simulink model "callZumoExtrinsic_runMotors"  (R2014a)
settings: Solver=FixedStepDiscrete  StartTime=0.0  StopTime=inf  FixedStep=0.1  RelTol=1e-3
settings Model: Creator=nrattner  LastModifiedBy=sandip

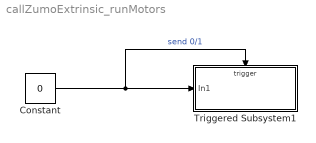
== system callZumoExtrinsic_runMotors ==
  Constant : Constant  Value=0
  Triggered Subsystem1 : Subsystem  TreatAsAtomicUnit=on
  wires:
  Constant/1 -> Triggered Subsystem1/Trigger, Triggered Subsystem1/1(In1)  "send 0/1"

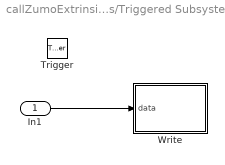
== system callZumoExtrinsic_runMotors/Triggered Subsystem1 ==
  In1 : Inport
  Trigger : TriggerPort  TriggerType=either  PortDimensions=1
  Write : MATLAB Function  TreatAsAtomicUnit=on
  wires:
  In1/1 -> Write/1(data)

== matlab function callZumoExtrinsic_runMotors/Triggered Subsystem1/Write ==
  data: data input
function write(data)
%#codegen

coder.extrinsic('comms.writeZumoBluetooth')
comms.writeZumoBluetooth(data);
